simulink model "SympatheticCurrent_Series"  (R2015a)
settings: Solver=ode45  StartTime=0.0  StopTime=2  RelTol=1e-3
undefined symbols (not defined in the file or in its folder): D11, Delta
libraries: powerlib x13
settings Model: Creator=baishuhua  LastModifiedBy=baishuhua
settings DebuggingCC: AlgebraicLoopMsg=none

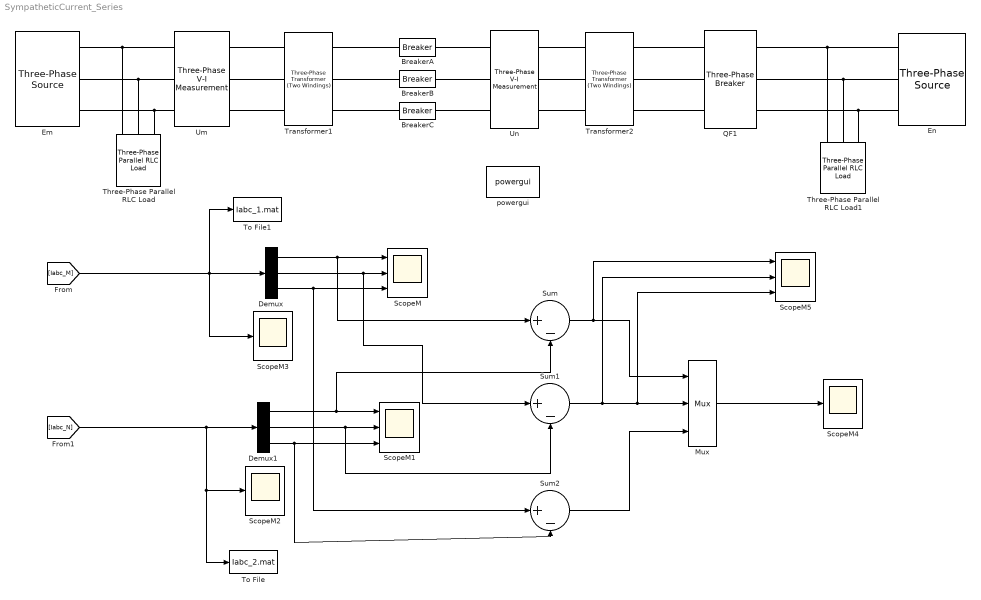
== system SympatheticCurrent_Series ==
  BreakerA : powerlib/Elements/Breaker  InitialState=0  SwitchingTimes=[1.1 2]  External=off  BreakerResistance=0.01  SnubberResistance=1e6  SnubberCapacitance=inf  Measurements=None  MoreParameters=on  NoBreakLoop=off
  BreakerB : powerlib/Elements/Breaker  InitialState=0  SwitchingTimes=[1.2 2]  External=off  BreakerResistance=0.01  SnubberResistance=1e6  SnubberCapacitance=inf  Measurements=None  MoreParameters=on  NoBreakLoop=off
  BreakerC : powerlib/Elements/Breaker  InitialState=0  SwitchingTimes=[1.3 2]  External=off  BreakerResistance=0.01  SnubberResistance=1e6  SnubberCapacitance=inf  Measurements=None  MoreParameters=on  NoBreakLoop=off
  Demux : Demux  Outputs=3
  Demux1 : Demux  Outputs=3
  Em : powerlib/Electrical Sources/Three-Phase Source  Voltage=35e3  PhaseAngle=180  Frequency=50  InternalConnection=Yg  SpecifyImpedance=off  Resistance=2.8929*1  Inductance=0.05*1  ShortCircuitLevel=100e6  BaseVoltage=35e3  XRratio=7  BusType=swing  Pref=0  Qref=0  Qmin=-inf  Qmax=inf
  En : powerlib/Electrical Sources/Three-Phase Source  Voltage=500e3  PhaseAngle=10  Frequency=50  InternalConnection=Yg  SpecifyImpedance=off  Resistance=0.8929  Inductance=16.58e-3  ShortCircuitLevel=100e6  BaseVoltage=500e3  XRratio=7  BusType=swing  Pref=0  Qref=0  Qmin=-inf  Qmax=inf
  Mux : Mux  Inputs=3
  QF1 : powerlib/Elements/Three-Phase Breaker  InitialState=open  SwitchA=on  SwitchB=on  SwitchC=on  SwitchTimes="[10.5  20]"  External=off  BreakerResistance=0.01  SnubberResistance=1e6  SnubberCapacitance=inf  Measurements=None
  ScopeM : Scope  NumInputPorts=3
      settings: ShowLegends=on  TimeRange=2  YMin=-500~-4000~-1750  YMax=4000~500~250  SampleInput=on
  ScopeM1 : Scope  NumInputPorts=3
      settings: ShowLegends=on  TimeRange=2  YMin=-500~-4000~-1750  YMax=4000~500~250  SampleInput=on
  ScopeM2 : Scope
      settings: ShowLegends=on  TimeRange=2  YMin=-500  YMax=4000  SaveName=ScopeData2  SampleInput=on
  ScopeM3 : Scope
      settings: ShowLegends=on  TimeRange=2  YMin=-500  YMax=4000  SaveName=ScopeData3  SampleInput=on
  ScopeM4 : Scope
      settings: ShowLegends=on  TimeRange=2  YMin=-500  YMax=4000  SaveName=ScopeData4  SampleInput=on
  ScopeM5 : Scope  NumInputPorts=3
      settings: ShowLegends=on  TimeRange=2  YMin=-500~-5~-5  YMax=4000~5~5  SaveName=ScopeData5  SampleInput=on
  Sum : Sum  Inputs=|+-
  Sum1 : Sum  Inputs=|+-
  Sum2 : Sum  Inputs=|+-
  Three-Phase Parallel RLC Load : powerlib/Elements/Three-Phase Parallel RLC Load  LConnTagsString=A|B|C  Configuration=Y (grounded)  NominalVoltage=35e3  NominalFrequency=50  ActivePower=30e6  InductivePower=0  CapacitivePower=1e6  Measurements=None  LoadType=constant PQ
  Three-Phase Parallel RLC Load1 : powerlib/Elements/Three-Phase Parallel RLC Load  LConnTagsString=A|B|C  Configuration=Y (grounded)  NominalVoltage=500e3  NominalFrequency=50  ActivePower=30e6  InductivePower=0  CapacitivePower=1e6  Measurements=None  LoadType=constant PQ
  To File : ToFile  Filename=Iabc_2.mat  MatrixName=Iabc_2  SaveFormat=Timeseries
  To File1 : ToFile  Filename=Iabc_1.mat  MatrixName=Iabc_1  SaveFormat=Timeseries
  Transformer1 : powerlib/Elements/Three-Phase Transformer (Two Windings)  Winding1Connection=Delta (D11)  Winding2Connection=Delta (D11)  CoreType=Three single-phase transformers  SetSaturation=on  Hysteresis=off  DataFile='hysteresis'  SetInitialFlux=on  Measurements=None  UNITS=pu  NominalPower=[ 300e6 , 50 ]  Winding1=[ 35e3 , 0.002 , 0.08 ]  Winding2=[ 220e3 , 0.002 , 0.08 ]  Rm=500  Lm=500  L0=0.5  Saturation=[ 0,0 ; 0.0024,1.2 ; 1.0,1.52 ]  InitialFluxes=[0.5 0 0]  MoreParameters=off  BreakLoop=off  DataType=off  TransfoNumber=1
  Transformer2 : powerlib/Elements/Three-Phase Transformer (Two Windings)  Winding1Connection=Delta (D11)  Winding2Connection=Delta (D11)  CoreType=Three single-phase transformers  SetSaturation=on  Hysteresis=off  DataFile='hysteresis'  SetInitialFlux=on  Measurements=None  UNITS=pu  NominalPower=[ 300e6 , 50 ]  Winding1=[ 220e3 , 0.002 , 0.08 ]  Winding2=[ 500e3 , 0.002 , 0.08 ]  Rm=500  Lm=500  L0=0.5  Saturation=[ 0,0 ; 0.0024,1.2 ; 1.0,1.52 ]  InitialFluxes=[0.7 -0.7 -0.7]  MoreParameters=off  BreakLoop=off  DataType=off  TransfoNumber=1
  Um : powerlib/Measurements/Three-Phase V-I Measurement  VoltageMeasurement=no  SetLabelV=on  LabelV=Vabc_M  Vpu=off  VpuLL=off  CurrentMeasurement=yes  SetLabelI=on  LabelI=Iabc_M  Ipu=on  Pbase=300e6  Vbase=35e3  OutputType=Complex  PhasorSimulation=off  PSBequivalent=0
  Un : powerlib/Measurements/Three-Phase V-I Measurement  VoltageMeasurement=no  SetLabelV=on  LabelV=Vabc_N  Vpu=off  VpuLL=off  CurrentMeasurement=yes  SetLabelI=on  LabelI=Iabc_N  Ipu=on  Pbase=300e6  Vbase=220e3  OutputType=Complex  PhasorSimulation=off  PSBequivalent=0
  powergui : powerlib/powergui  Priority=1  SimulationMode=Discrete  SolverType=Tustin/Backward Euler (TBE)  SampleTime=1e-4  frequency=60  SPID=off  DisableSnubberDevices=off  DisableRonSwitches=off  DisableVfSwitches=off  SwTol=0  DisplayEquations=off  Interpol=off  methode=off  Ts=100  FunctionMessages=off  echomessages=off  HookPort=off  EnableUseOfTLC=off  x0status=blocks  frequencyindice=50  Pbase=100e6  ErrMax=1e-4  Iterations=50  UnitsV=kV  UnitsW=MW  buscounter=0  RestoreLinks=warning  ResistiveCurrentMeasurement=off  Frange=[0:2:500]  Ylog=off  Xlog=on  ShowGrid=off  save=off  variable=ZData  structure=0  ZoomFFT=off  StartTime=0.0  cycles=1  DisplayStyle=1  fundamental=60  FreqAxis=off  MaxFrequency=1000  frequencyindicesteady=1  RmsSteady=1  display=off
  wires:
  [Iabc_M] -> To File1/1, ScopeM3/1, Demux/1
  Demux/1 -> Sum/1, ScopeM/1
  Demux/2 -> Sum1/1, ScopeM/2
  Demux/3 -> Sum2/1, ScopeM/3
  Demux1/1 -> Sum/2, ScopeM1/1
  Demux1/2 -> Sum1/2, ScopeM1/2
  Demux1/3 -> Sum2/2, ScopeM1/3
  Sum/1 -> ScopeM5/1, Mux/1
  Sum1/1 -> ScopeM5/2, ScopeM5/3, Mux/2
  Sum2/1 -> Mux/3
  Mux/1 -> ScopeM4/1
  [Iabc_N] -> To File/1, ScopeM2/1, Demux1/1
  connections:
  Em/RConn1 -- Three-Phase Parallel RLC Load/LConn1 -- Um/LConn1
  Em/RConn2 -- Um/LConn2 -- Three-Phase Parallel RLC Load/LConn2
  Em/RConn3 -- Um/LConn3 -- Three-Phase Parallel RLC Load/LConn3
  Three-Phase Parallel RLC Load1/LConn1 -- En/RConn1 -- QF1/RConn1
  Three-Phase Parallel RLC Load1/LConn2 -- En/RConn2 -- QF1/RConn2
  Three-Phase Parallel RLC Load1/LConn3 -- QF1/RConn3 -- En/RConn3
  BreakerA/LConn1 -- Transformer1/RConn1
  BreakerB/LConn1 -- Transformer1/RConn2
  BreakerC/LConn1 -- Transformer1/RConn3
  Transformer1/LConn1 -- Um/RConn1
  Transformer1/LConn3 -- Um/RConn3
  Transformer1/LConn2 -- Um/RConn2
  BreakerA/RConn1 -- Un/LConn1
  BreakerB/RConn1 -- Un/LConn2
  BreakerC/RConn1 -- Un/LConn3
  Transformer2/LConn1 -- Un/RConn1
  Transformer2/LConn2 -- Un/RConn2
  Transformer2/LConn3 -- Un/RConn3
  QF1/LConn1 -- Transformer2/RConn1
  QF1/LConn2 -- Transformer2/RConn2
  QF1/LConn3 -- Transformer2/RConn3
